simulink subsystem "accelerometer"  (R2024b)
settings: Solver=VariableStepAuto  StartTime=0.0  StopTime=10.0  RelTol=1e-3
undefined symbols (not defined in the file or in its folder): GRAVITY, observer_rate
settings Model: Creator=yevge  LastModifiedBy=yevge

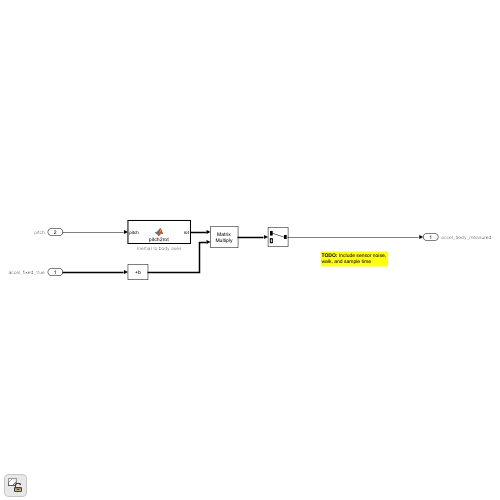
[thumbnail: Simulink's stored preview of the top-level diagram]
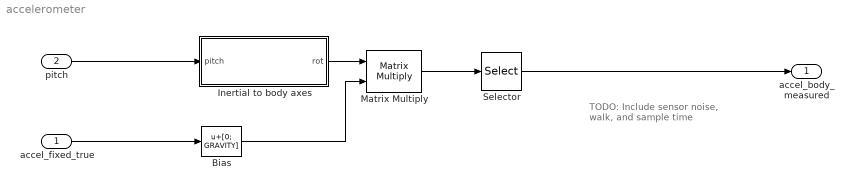
== system accelerometer ==
  note: TODO: Include sensor noise, walk, and sample time
  accel_fixed_true : Inport  Unit=m/s^2  PortDimensions=[2 1]
  pitch : Inport  Port=2  Unit=rad  PortDimensions=1
  Bias : Bias  Bias=[0; GRAVITY]  SaturateOnIntegerOverflow=off
  Inertial to body axes : MATLAB Function  TreatAsAtomicUnit=on
  Matrix Multiply : Product  Multiplication=Matrix(*)
  Selector : Selector  InputPortWidth=2  IndexOptions=Index vector (dialog)  Indices=1  OutputSizes=1
  accel_body_measured : Outport  Unit=m/s^2  PortDimensions=1  SampleTime=1/observer_rate
  wires:
  pitch/1 -> Inertial to body axes/1(pitch)
  Inertial to body axes/1(rot) -> Matrix Multiply/1
  accel_fixed_true/1 -> Bias/1
  Matrix Multiply/1 -> Selector/1
  Bias/1 -> Matrix Multiply/2
  Selector/1 -> accel_body_measured/1

== matlab function accelerometer/Inertial to body axes ==
  data: pitch input size=1; rot output size=[2 2]
function rot = pitch2rot(pitch)
    ct = cos(pitch);
    st = sin(pitch);
    rot = [ct st
        -st ct];
end
